simulink library "getTargetPoint"  (R2018a)
settings: Solver=VariableStepAuto  StartTime=0.0  StopTime=10.0  RelTol=1e-3
undefined symbols (not defined in the file or in its folder): iterationPhase_enum
libraries: calculateTargetWaypointReelIn x1, calculateTargetWaypointReelIn_cl x1, simulink x1
settings Model: Creator=mitch  LastModifiedBy=mitch

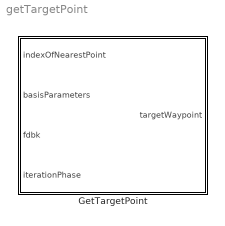
== system getTargetPoint ==
  GetTargetPoint : Subsystem

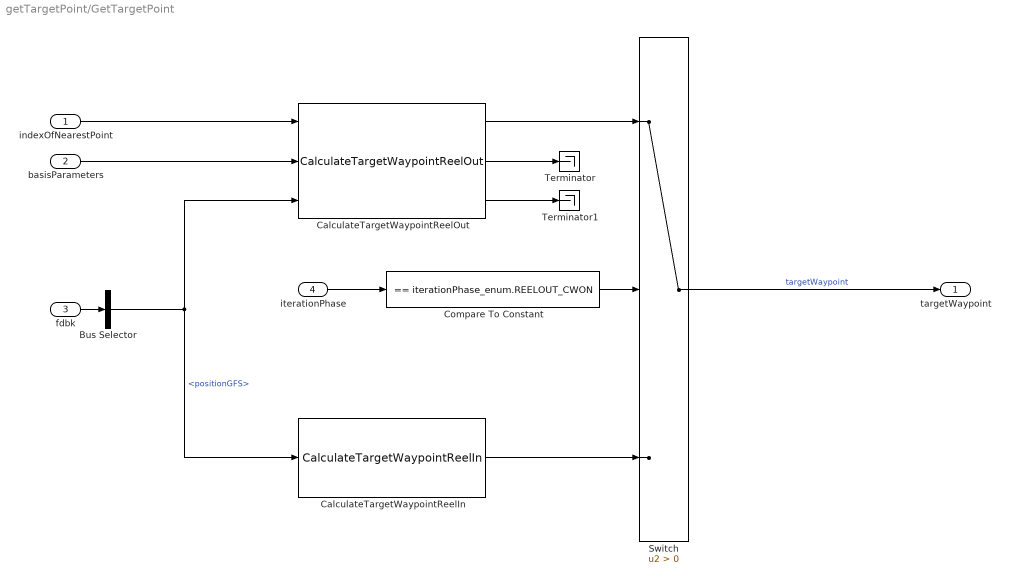
== system getTargetPoint/GetTargetPoint ==
  indexOfNearestPoint : Inport
  basisParameters : Inport  Port=2
  fdbk : Inport  Port=3  OutDataTypeStr=Bus: busPlantFeedback
  iterationPhase : Inport  Port=4
  Bus Selector : BusSelector  OutputSignals=positionGFS
  CalculateTargetWaypointReelIn : calculateTargetWaypointReelIn/CalculateTargetWaypointReelIn
  CalculateTargetWaypointReelOut : calculateTargetWaypointReelIn_cl/CalculateTargetWaypointReelOut
  Compare To Constant : simulink/Logic and Bit Operations/Compare To Constant  relop===  const=iterationPhase_enum.REELOUT_CWON  OutDataTypeStr=boolean
  Switch : Switch  Criteria=u2 > Threshold
  Terminator : Terminator
  Terminator1 : Terminator
  targetWaypoint : Outport
  wires:
  fdbk/1 -> Bus Selector/1
  indexOfNearestPoint/1 -> CalculateTargetWaypointReelOut/1
  basisParameters/1 -> CalculateTargetWaypointReelOut/2
  Bus Selector/1 -> CalculateTargetWaypointReelIn/1, CalculateTargetWaypointReelOut/3  "<positionGFS>"
  iterationPhase/1 -> Compare To Constant/1
  Compare To Constant/1 -> Switch/2
  Switch/1 -> targetWaypoint/1  "targetWaypoint"
  CalculateTargetWaypointReelOut/2 -> Terminator/1
  CalculateTargetWaypointReelOut/3 -> Terminator1/1
  CalculateTargetWaypointReelOut/1 -> Switch/1
  CalculateTargetWaypointReelIn/1 -> Switch/3
